simulink model "serial_2_test"  (R2022a)
settings: Solver=FixedStepAuto  StartTime=0.0  StopTime=10.0  FixedStep=1e-3  RelTol=1e-3  EnableMultiTasking=on
libraries: frdmk64flib x3
settings Model: ExtModeTrigDuration=5  Creator=liaml  LastModifiedBy=liaml
settings OptimizationCC: EnhancedBackFolding=on  PassReuseOutputArgsAs=Individual arguments  ZeroExternalMemoryAtStartup=off  ZeroInternalMemoryAtStartup=off  MaxStackSize=64  OptimizeBlockOrder=speed  DifferentSizesBufferReuse=on  OptimizationCustomize=off  EfficientTunableParamExpr=on
settings DebuggingCC: ParameterTunabilityLossMsg=error
settings HardwareCC: ProdBitPerPointer=32  ProdBitPerSizeT=32  ProdBitPerPtrDiffT=32  ProdLargestAtomicInteger=Long  ProdLargestAtomicFloat=Double  ProdWordSize=32  ProdHWDeviceType=ARM Compatible->ARM Cortex
settings SFSimCC: MATLABDynamicMemAlloc=off
settings RTWCC: SystemTargetFile=ert.tlc  HardwareBoard=NXP FRDM-K64F  TLCOptions="-aInlineSetEventsForThisBaseRateFcn=TLC_FALSE -aSuppressMultiTaskScheduler=TLC_FALSE  -aRateBasedStepFcn=0"  TemplateMakefile=ert_default_tmf  Toolchain=GNU Tools for ARM Embedded Processors
settings CodeAppCC: ForceParamTrailComments=on  IgnoreCustomStorageClasses=off  OperatorAnnotations=on  SimulinkDataObjDesc=on  SFDataObjDesc=on  InsertBlockDesc=on
settings ERTTargetCC: ExtModeTransport=4  ExtModeMexFile=sendToCommService

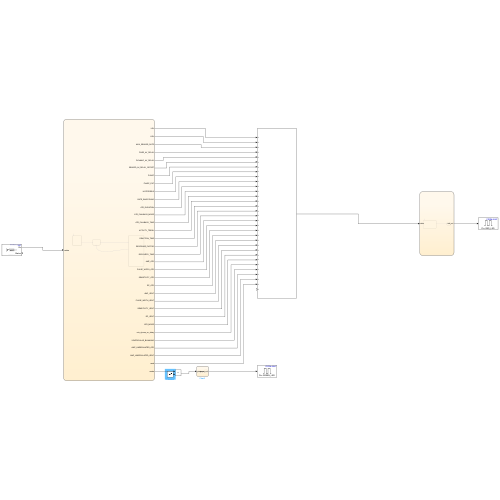
[thumbnail: Simulink's stored preview of the top-level diagram]
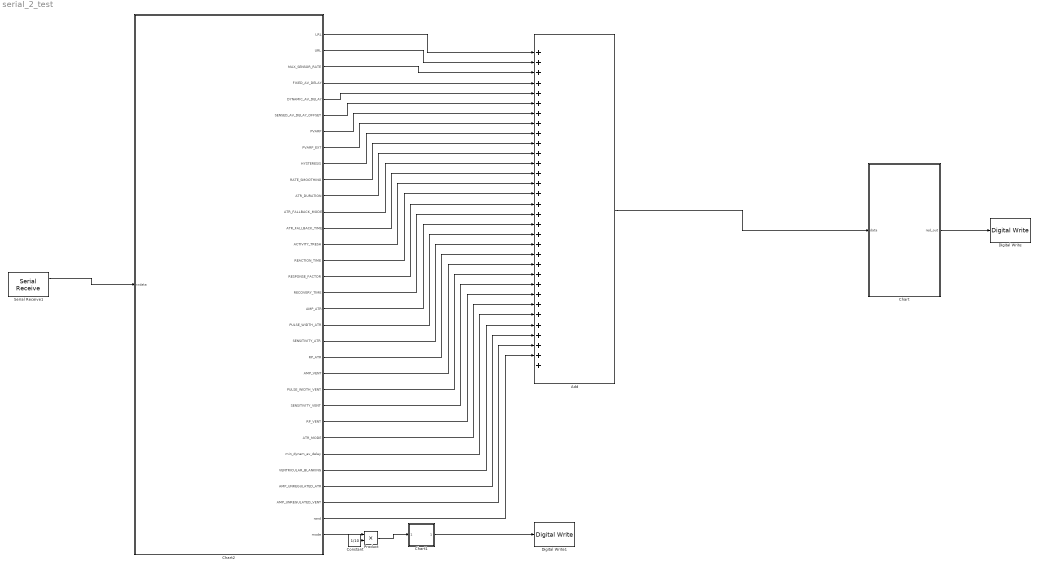
== system serial_2_test ==
  Add : Sum  Inputs=++++++++++++++++++++++++++++++++
  Chart : Stateflow chart  TreatAsAtomicUnit=on
  Chart1 : Stateflow chart  TreatAsAtomicUnit=on
  Chart2 : Stateflow chart  TreatAsAtomicUnit=on
  Constant : Constant  Value=1/10
  Digital Write : frdmk64flib/Digital Write  Whichpin=RED_LED
  Digital Write1 : frdmk64flib/Digital Write  Whichpin=GREEN_LED
  Product : Product
  Serial Receive1 : frdmk64flib/Serial Receive  SCIModule=0  Baudrate=uint32(9600)  Parity=None  StopBits=1  HardwareFlowControl=None  ByteOrder=LittleEndian  DataType=int8  DataLength=37  BlockingMode=off  OutputStatus=on  SampleTime=-1
  wires:
  Serial Receive1/1 -> Chart2/1(rxdata)
  Add/1 -> Chart/1(data)
  Chart/1(red_out) -> Digital Write/1
  Chart2/1(LRL) -> Add/1
  Chart2/2(URL) -> Add/2
  Chart2/3(MAX_SENSOR_RATE) -> Add/3
  Chart2/4(FIXED_AV_DELAY) -> Add/4
  Chart2/5(DYNAMIC_AV_DELAY) -> Add/5
  Chart2/6(SENSED_AV_DELAY_OFFSET) -> Add/6
  Chart2/7(PVARP) -> Add/7
  Chart2/8(PVARP_EXT) -> Add/8
  Chart2/9(HYSTERESIS) -> Add/9
  Chart2/10(RATE_SMOOTHING) -> Add/10
  Chart2/11(ATR_DURATION) -> Add/11
  Chart2/12(ATR_FALLBACK_MODE) -> Add/12
  Chart2/13(ATR_FALLBACK_TIME) -> Add/13
  Chart2/14(ACTIVITY_TRESH) -> Add/14
  Chart2/15(REACTION_TIME) -> Add/15
  Chart2/16(RESPONSE_FACTOR) -> Add/16
  Chart2/17(RECOVERY_TIME) -> Add/17
  Chart2/18(AMP_ATR) -> Add/18
  Chart2/19(PULSE_WIDTH_ATR) -> Add/19
  Chart2/20(SENSITIVITY_ATR) -> Add/20
  Chart2/21(RP_ATR) -> Add/21
  Chart2/22(AMP_VENT) -> Add/22
  Chart2/23(PULSE_WIDTH_VENT) -> Add/23
  Chart2/24(SENSITIVITY_VENT) -> Add/24
  Chart2/25(RP_VENT) -> Add/25
  Chart2/26(ATR_MODE) -> Add/26
  Chart2/27(min_dynam_av_delay) -> Add/27
  Chart2/28(VENTRICULAR_BLANKING) -> Add/28
  Chart2/29(AMP_UNREGULATED_ATR) -> Add/29
  Chart2/30(AMP_UNREGULATED_VENT) -> Add/30
  Chart2/31(rand) -> Add/31
  Chart2/32(mode) -> Product/1
  Product/1 -> Chart1/1(green_en)
  Chart1/1(green_out) -> Digital Write1/1
  Constant/1 -> Product/2

== stateflow chart serial_2_test/Chart2 ==
  state SET_PRAMS
    entry:
    rand = 0;
    mode = typecast(rxdata(1),'int8');
    LRL =  typecast(rxdata(2),'int8');
    URL = typecast(rxdata(3),'int8');
    MAX_SENSOR_RATE =  typecast(rxdata(4),'int8');
    FIXED_AV_DELAY =  typecast(rxdata(5),'int8');
    DYNAMIC_AV_DELAY =  typecast(rxdata(6),'int8');
    min_dynam_av_delay = typecast(rxdata(7),'int8');
    SENSED_AV_DELAY_OFFSET =typecast(rxdata(8),'int8');
    PVARP = typecast(rxdata(9),'int8');
    PVARP_EXT = typecast(rxdata(10),'int8');
    HYSTERESIS = typecast(rxdata(11),'int8');
    RATE_SMOOTHING = typecast(rxdata(12),'int8');
    ATR_MODE = typecast(rxdata(13),'int8');
    ATR_DURATION = typecast(rxdata(14),'int8');
    ATR_FALLBACK_MODE =typecast(rxdata(15),'int8');
    ATR_FALLBACK_TIME = typecast(rxdata(16),'int8');
    VENTRICULAR_BLANKING =typecast(rxdata(17),'int8');
    ACTIVITY_TRESH =typecast(rxdata(18),'int8');
    REACTION_TIME = typecast(rxdata(19),'int8');
    RESPONSE_FACTOR =typecast(rxdata(20),'int8');
    RECOVERY_TIME = typecast(rxdata(21),'int8');
    AMP_ATR =typecast(rxdata(22),'int8');
    AMP_UNREGULATED_ATR =typecast(rxdata(23),'int8');
    PULSE_WIDTH_ATR=typecast(rxdata(24),'int8');
    SENSITIVITY_ATR =typecast(rxdata(25),'int8');
    RP_ATR = typecast(rxdata(26),'int8');
    AMP_ATR =typecast(rxdata(27),'int8');
    AMP_UNREGULATED_ATR =typecast(rxdata(28),'int8');
    PULSE_WIDTH_ATR=typecast(rxdata(29),'int8');
    SENSITIVITY_ATR =typecast(rxdata(30),'int8');
    RP_ATR = typecast(rxdata(31),'int8');
    AMP_VENT =typecast(rxdata(32),'int8');
    AMP_UNREGULATED_VENT =typecast(rxdata(33),'int8');
    PULSE_WIDTH_VENT=typecast(rxdata(34),'int8');
    SENSITIVITY_VENT = typecast(rxdata(35),'int8');
    RP_VENT =typecast(rxdata(36),'int8');
  state Init
    entry:
  state STANDBY
  (default) -> Init
  Init -> STANDBY
  STANDBY -> SET_PRAMS : [rxdata(37) == hex2dec('21')]
  SET_PRAMS -> STANDBY
  data: rxdata input; LRL output size=1; URL output size=1; MAX_SENSOR_RATE output size=1; FIXED_AV_DELAY output size=1; DYNAMIC_AV_DELAY output size=1; SENSED_AV_DELAY_OFFSET output size=1; PVARP output size=1; PVARP_EXT output size=1; HYSTERESIS output size=1; RATE_SMOOTHING output size=1; ATR_DURATION output size=1; ATR_FALLBACK_MODE output size=1; ATR_FALLBACK_TIME output size=1; ACTIVITY_TRESH output size=1; REACTION_TIME output size=1; RESPONSE_FACTOR output size=1; RECOVERY_TIME output size=1; AMP_ATR output size=1; PULSE_WIDTH_ATR output size=1; SENSITIVITY_ATR output size=1; RP_ATR output size=1; AMP_VENT output size=1; PULSE_WIDTH_VENT output size=1; SENSITIVITY_VENT output size=1; RP_VENT output size=1; ATR_MODE output size=1; min_dynam_av_delay output size=1; VENTRICULAR_BLANKING output size=1; AMP_UNREGULATED_ATR output size=1; AMP_UNREGULATED_VENT output size=1; rand output size=1; mode output size=1

== stateflow chart serial_2_test/Chart1 ==
  state green_on
    entry:
    green_out = true;
  state init
    entry:
  (default) -> init
  init -> green_on : [green_en == 10]
  data: green_en input; green_out output

== stateflow chart serial_2_test/Chart ==
  state Init
    entry:
    red_out = false;
  state RED_ON
    entry:
    red_out= true;
  (default) -> Init
  Init -> RED_ON : [data == 31]
  data: data input; red_out output
